simulink library "gravity_field_lib"  (R2016b)
settings: Solver=VariableStepAuto  StartTime=0.0  StopTime=10.0  RelTol=1e-3
undefined symbols (not defined in the file or in its folder): sim_params
libraries: eci_to_body x1
settings Model: Creator=bbarz_000  LastModifiedBy=taylorreynolds
settings OptimizationCC: LifeSpan=inf
settings DebuggingCC: SFExecutionAtInitializationDiag=none

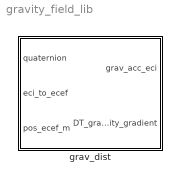
== system gravity_field_lib ==
  grav_dist : Subsystem

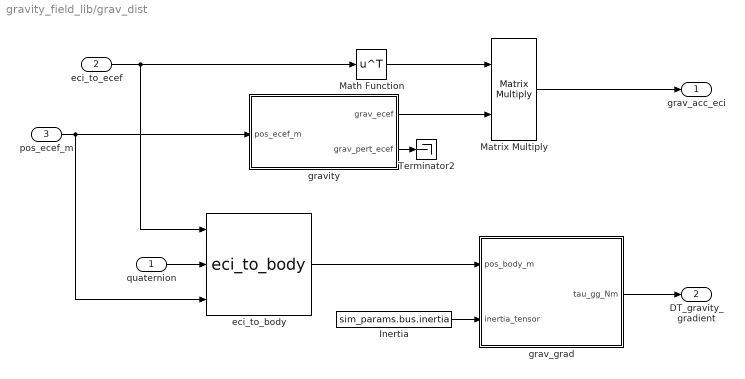
== system gravity_field_lib/grav_dist ==
  quaternion : Inport
  eci_to_ecef : Inport  Port=2
  pos_ecef_m : Inport  Port=3
  Inertia : Constant  Value=sim_params.bus.inertia
  Math Function : Math  Operator=transpose  SaturateOnIntegerOverflow=on
  Matrix Multiply : Product  Multiplication=Matrix(*)
  Terminator2 : Terminator
  eci_to_body : eci_to_body/eci_to_body
  grav_grad : MATLAB Function  TreatAsAtomicUnit=on
  gravity : MATLAB Function  TreatAsAtomicUnit=on
  grav_acc_eci : Outport
  DT_gravity_gradient : Outport  Port=2
  wires:
  Math Function/1 -> Matrix Multiply/1
  gravity/1(grav_ecef) -> Matrix Multiply/2
  gravity/2(grav_pert_ecef) -> Terminator2/1
  pos_ecef_m/1 -> eci_to_body/3, gravity/1(pos_ecef_m)
  eci_to_ecef/1 -> eci_to_body/1, Math Function/1
  Inertia/1 -> grav_grad/2(inertia_tensor)
  eci_to_body/1 -> grav_grad/1(pos_body_m)
  grav_grad/1(tau_gg_Nm) -> DT_gravity_gradient/1
  Matrix Multiply/1 -> grav_acc_eci/1
  quaternion/1 -> eci_to_body/2

== matlab function gravity_field_lib/grav_dist/gravity ==
  data: pos_ecef_m input; grav_ecef output; grav_pert_ecef output
function [grav_ecef, grav_pert_ecef] = grav(pos_ecef_m)
% HuskySat-1, ADCS Subsystem
% Last Update: T. Reynolds - 12.7.17

% calculates acceleration from Earth (incl. oblateness)

% constants
Req = 6.378137e6;             % [m] Earth equator radius
J2 = 1.08262668355e-3;           % gravitational perturbation parameter 
J3 = -2.53265648533e-6;
J4 = -1.61962159137e-6;
% J5 = -2.27296082869e-7;
% J6 = 5.40681239107e-7;
mu = 3.986004418e14; % [m3/s2] 

% position vector components
rX = pos_ecef_m(1);
rY = pos_ecef_m(2);
rZ = pos_ecef_m(3);

% mag. of position vector
r = norm(pos_ecef_m);

accel = zeros(3,4);
% point-mass effect
accel(:,1) = -mu/r^2*[  rX/r;
                        rY/r;
                        rZ/r];

% oblateness effects (J2 through J6 perturbations)
% Fundamentals of ADCS (Junkins & Markley)
accel(:,2) = -3/2*J2*(mu/r^2)*(Req/r)^2*[   (1 - 5*(rZ/r)^2)*rX/r;
                                            (1 - 5*(rZ/r)^2)*rY/r;
                                            (3 - 5*(rZ/r)^2)*rZ/r];

accel(:,3) = -1/2*J3*(mu/r^2)*(Req/r)^3*[   5*(7*(rZ/r)^3 - 3*(rZ/r))*rX/r;
                                            5*(7*(rZ/r)^3 - 3*(rZ/r))*rY/r;
                                            3*(10*(rZ/r)^2 - 35/3*(rZ/r)^4 - 1)];
                                
accel(:,4) = -5/8*J4*(mu/r^2)*(Req/r)^4*[   (3 - 42*(rZ/r)^2 + 63*(rZ/r)^4)*rX/r;
                                            (3 - 42*(rZ/r)^2 + 63*(rZ/r)^4)*rY/r;
                                            -(15 - 70*(rZ/r)^2 + 63*(rZ/r)^4)*rZ/r];
                                
% accel(:,5) = -1/8*J5*(mu/r^2)*(Req/r)^5*[   3*(35*(rZ/r) - 210*(rZ/r)^3 + 231*(rZ/r)^5)*rX/r;
%                                             3*(35*(rZ/r) - 210*(rZ/r)^3 + 231*(rZ/r)^5)*rY/r;
%                                             (15 - 315*(rZ/r)^2 + 945*(rZ/r)^4 - 693*(rZ/r)^6)];
%                                 
% accel(:,6) = 1/16*J6*(mu/r^2)*(Req/r)^6*[   (35 - 945*(rZ/r)^2 + 3465*(rZ/r)^4 - 3003*(rZ/r)^6)*rX/r;
%                                             (35 - 945*(rZ/r)^2 + 3465*(rZ/r)^4 - 3003*(rZ/r)^6)*rY/r;
%                                             (2205*(rZ/r)^2 - 4851*(rZ/r)^4 + 3003*(rZ/r)^6 - 315)*rZ/r];

grav_ecef = sum(accel, 2);
grav_pert_ecef = sum(accel(:,2:4), 2);

== matlab function gravity_field_lib/grav_dist/grav_grad ==
  data: pos_body_m input; tau_gg_Nm output; inertia_tensor input
function tau_gg_Nm = grav_grad(pos_body_m, inertia_tensor)
%#codegen
% HuskySat-1, ADCS Subsystem
% Last Update: T. Reynolds - 12.5.17
%
% Computes the gravity gradient torque on the s/c.
%   Reference: dR-D-F, Spacecraft Dynamics & Control: An Intro, 2013.

MU = 3.986004418e14; % m3/s2

a   = pos_body_m;
b   = inertia_tensor*pos_body_m;

axb     = skew(a)*b;

tau_gg_Nm = 3*MU/(norm(a)^5)*axb; % Nm

end

function Sa     = skew( a )
a1   = a(1);
a2   = a(2);
a3   = a(3);

Sa  = [ 0      -a3     a2;
        a3      0     -a1;
       -a2      a1     0 ];

end
